simulink model "IEEE39bus"  (Simulink 8.5)
settings: Solver=ode3  SolverMode=SingleTasking  StartTime=0.0  StopTime=50  FixedStep=Ts  RelTol=1e-3
PostLoadFcn:
  | Ts=25e-6; IEEE39BusLineLength;
  | vNomHV = 345E3;fNom=50;load('Dynamicload.mat');
InitFcn:
  | Ts=25e-6; IEEE39BusLineLength;
  | vNomHV = 345E3;fNom=50;load('Dynamicload.mat');
undefined symbols (not defined in the file): D1, Delta, load15, load16, load18, load20, load21, load23, load24, load25, load26, load27, load28, load29, load3, load39, load4, load7, load8, TL_10_11_len, TL_10_13_len, TL_13_14_len, TL_14_15_len, TL_15_16_len, TL_16_17_len, TL_16_19_len, TL_16_21_len, TL_16_24_len, TL_17_18_len, TL_17_27_len, TL_1_2_len, TL_1_39_len, TL_21_22_len, TL_22_23_len, TL_24_23_len, TL_25_26_len, TL_26_27_len, TL_26_28_len, TL_26_29_len, TL_28_29_len, TL_2_25_len, TL_2_2_len, TL_3_18_len, TL_3_4_len, TL_4_14_len, TL_4_5_len, TL_5_6_len, TL_5_8_len, TL_6_11_len, TL_6_7_len, TL_7_8_len, TL_8_9_len, TL_9_39_len
libraries: powerlib x175, op_dpl_lib x34, rtlab x14, sps_avr x9, powerlib_extras x2, artemis x1, powerlib_meascontrol x1
(part 4 of 5)

== system IEEE39bus/SS_WestSystem1/GT 1  ==
  The Electric Power Grid : Subsystem  mask(The Electric Power Grid){pTotal=3, fNom=50, vNom=22e3*(1E-3)*1.05, pFeeder=185.5-50}
      mask prompts: pTotal "Total grid generation (GWatt)"; fNom "Nominal frequency (Hz)"; vNom "Nominal L-L voltage (kV)"; pFeeder "Initial feeder consumption (MWatt)"
      mask init:
      | % this is a patch for Simulink limitation on expression evaluation at model
      | % opening to avoid a error message
      | initPm0=(0.7*pTotal*1E9+pFeeder*1E6+1E6)/(pTotal*1E9);
      mask Display: image(imread('EPG.jpg'))
  A : PMIOPort  Port=1  Side=Right
  B : PMIOPort  Port=2  Side=Right
  C : PMIOPort  Port=3  Side=Right
  tag scope: V_G1=global
  wires:
  [V_bus_G1] -> [V_G1]
  connections:
  The Electric Power Grid/RConn3 -- C/RConn1
  B/RConn1 -- The Electric Power Grid/RConn2
  A/RConn1 -- The Electric Power Grid/RConn1

== system IEEE39bus/SS_WestSystem1/Load 39 ==
  Bus_L39 : powerlib/Measurements/Three-Phase V-I Measurement  VoltageMeasurement=phase-to-ground  SetLabelV=off  LabelV=V_Bus_L39  Vpu=off  VpuLL=off  CurrentMeasurement=yes  SetLabelI=on  LabelI=I_L39  Ipu=off  Pbase=100e6  Vbase=230e3  OutputType=Complex  PhasorSimulation=off  PSBequivalent=0
  Terminator : Terminator
  Three-Phase Dynamic Load : powerlib/Elements/Three-Phase Dynamic Load  NominalVoltage=[345e3 50 ]  ActiveReactivePowers=[1.104e+09 2.5e+08]  PositiveSequence=[1.02945 21.8447]  ExternalControl=on  NpNq=[0 0]  TimeConstants="[0  0  0  0]"  MinimumVoltage=0.7  LoadFlowParameters=[4,0,0,0,0]
  A : PMIOPort  Port=1  Side=Left
  B : PMIOPort  Port=2  Side=Left
  C : PMIOPort  Port=3  Side=Left
  tag scope: V_L39=global
  wires:
  Three-Phase Dynamic Load/1 -> Terminator/1
  Bus_L39/1 -> [V_L39]
  [load39] -> Three-Phase Dynamic Load/1
  connections:
  Three-Phase Dynamic Load/LConn1 -- Bus_L39/RConn1
  C/RConn1 -- Bus_L39/LConn3
  B/RConn1 -- Bus_L39/LConn2
  A/RConn1 -- Bus_L39/LConn1
  Bus_L39/RConn2 -- Three-Phase Dynamic Load/LConn2
  Bus_L39/RConn3 -- Three-Phase Dynamic Load/LConn3

== system IEEE39bus/SS_WestSystem1/Load 4 ==
  Bus_L4 : powerlib/Measurements/Three-Phase V-I Measurement  VoltageMeasurement=phase-to-ground  SetLabelV=off  LabelV=V_Bus_L4  Vpu=off  VpuLL=off  CurrentMeasurement=yes  SetLabelI=on  LabelI=I_L4  Ipu=off  Pbase=100e6  Vbase=230e3  OutputType=Complex  PhasorSimulation=off  PSBequivalent=0
  Terminator : Terminator
  Three-Phase Dynamic Load : powerlib/Elements/Three-Phase Dynamic Load  NominalVoltage=[ 345e3 50 ]  ActiveReactivePowers=[5e+08 1.84e+08]  PositiveSequence=[0.993488 19.1617]  ExternalControl=on  NpNq=[0 0]  TimeConstants="[0  0  0  0]"  MinimumVoltage=0.7  LoadFlowParameters=[4,0,0,0,0]
  A : PMIOPort  Port=1  Side=Left
  B : PMIOPort  Port=2  Side=Left
  C : PMIOPort  Port=3  Side=Left
  tag scope: V_L4=global
  wires:
  Three-Phase Dynamic Load/1 -> Terminator/1
  Bus_L4/1 -> [V_L4]
  [load4] -> Three-Phase Dynamic Load/1
  connections:
  Three-Phase Dynamic Load/LConn3 -- Bus_L4/RConn3
  Three-Phase Dynamic Load/LConn2 -- Bus_L4/RConn2
  A/RConn1 -- Bus_L4/LConn1
  B/RConn1 -- Bus_L4/LConn2
  C/RConn1 -- Bus_L4/LConn3
  Three-Phase Dynamic Load/LConn1 -- Bus_L4/RConn1

== system IEEE39bus/SS_WestSystem1/Load 8 ==
  Bus_L8 : powerlib/Measurements/Three-Phase V-I Measurement  VoltageMeasurement=phase-to-ground  SetLabelV=off  LabelV=V_Bus_L8  Vpu=off  VpuLL=off  CurrentMeasurement=yes  SetLabelI=on  LabelI=I_L8  Ipu=off  Pbase=100e6  Vbase=230e3  OutputType=Complex  PhasorSimulation=off  PSBequivalent=0
  Terminator : Terminator
  Three-Phase Dynamic Load : powerlib/Elements/Three-Phase Dynamic Load  NominalVoltage=[345e3 50 ]  ActiveReactivePowers=[5.22e+08 1.76e+08]  PositiveSequence=[0.991583 18.8054]  ExternalControl=on  NpNq=[0 0]  TimeConstants="[0  0  0  0]"  MinimumVoltage=0.7  LoadFlowParameters=[4,0,0,0,0]
  A : PMIOPort  Port=1  Side=Left
  B : PMIOPort  Port=2  Side=Left
  C : PMIOPort  Port=3  Side=Left
  tag scope: V_L8=global
  wires:
  Three-Phase Dynamic Load/1 -> Terminator/1
  Bus_L8/1 -> [V_L8]
  [load8] -> Three-Phase Dynamic Load/1
  connections:
  Three-Phase Dynamic Load/LConn1 -- Bus_L8/RConn1
  C/RConn1 -- Bus_L8/LConn3
  B/RConn1 -- Bus_L8/LConn2
  A/RConn1 -- Bus_L8/LConn1
  Three-Phase Dynamic Load/LConn2 -- Bus_L8/RConn2
  Three-Phase Dynamic Load/LConn3 -- Bus_L8/RConn3

== system IEEE39bus/SS_WestSystem1/Machines Measurements ==
  Mux1 : Mux
  Machines Measurements : Outport
  wires:
  Mux1/1 -> Machines Measurements/1
  [Wm_G1] -> Mux1/4
  [Q_G1] -> Mux1/3
  [P_G1] -> Mux1/2
  [V_G1] -> Mux1/1

== system IEEE39bus/SS_WestSystem2/Buses Current_W ==
  Mux3 : Mux  Inputs=6
  Current : Outport
  wires:
  Mux3/1 -> Current/1
  [I_bus_6] -> Mux3/1
  [I_L7] -> Mux3/2
  [I_bus_13] -> Mux3/6
  [I_L12] -> Mux3/5
  [I_bus_11] -> Mux3/4
  [I_bus_10] -> Mux3/3

== system IEEE39bus/SS_WestSystem2/Buses voltages_W ==
  Mux3 : Mux  Inputs=6
  Voltages : Outport
  wires:
  [V_L7] -> Mux3/2
  [V_bus_10] -> Mux3/3
  [V_L12] -> Mux3/5
  [V_bus_11] -> Mux3/4
  [V_bus_13] -> Mux3/6
  [V_bus_6] -> Mux3/1
  Mux3/1 -> Voltages/1

== system IEEE39bus/SS_WestSystem2/GT 2- Slack ==
  5 MW : powerlib/Elements/Three-Phase Parallel RLC Load  LConnTagsString=A|B|C  Configuration=Y (grounded)  NominalVoltage=22e3  NominalFrequency=50  ActivePower=5e6  InductivePower=0  CapacitivePower=0  Measurements=None  LoadType=constant Z
  Bus Selector1 : BusSelector  OutputSignals="dq0 components.Stator voltage  vq (pu),dq0 components.Stator voltage  vd (pu),Mechanical.Rotor speed  wm  (pu),Mechanical.Rotor speed deviation  dw (pu),Output active power   Peo (pu),Output reactive power  Qeo (pu)"
  Bus 31 : powerlib/Measurements/Three-Phase V-I Measurement  VoltageMeasurement=phase-to-ground  SetLabelV=on  LabelV=V_bus_G2  Vpu=off  VpuLL=off  CurrentMeasurement=no  SetLabelI=on  LabelI=I_bus_G2  Ipu=off  Pbase=100e6  Vbase=16.5e3  OutputType=Complex  PhasorSimulation=off  PSBequivalent=0
  Excitation System : sps_avr/Excitation System  tr=20e-3  reg=[ 200, 0.02 ]  exc=[ 1, 0 .19]  tgr=[ 0, 0 ]  damp=[ 0.0012, 1 ]  sat=[ 0, 0 ]  lim=[ 0, 7.32, 0 ]  v0=[0.982 2.0635]
  GT1_CB2 : Subsystem
  Ground : Ground
  HTG : powerlib/Machines/Hydraulic Turbine and Governor  sm="[ 10/3  0.07 ]"  gate="[  0.01  0.97518  -0.1  0.1 ]"  reg="[  0.05  1.163  0.105  0  0.01  ]"  hyd="[  0  2.67  ]"  dref=0  po=0.84
  Load 31 : Subsystem
  Load Flow Bus : powerlib/Measurements/Load Flow Bus  LConnTagsString=a  ID=Bus-31  Vbase=22000  Vref=0.982  Vangle=0  VLF=0.982  angleLF=0
      settings: AttributesFormatString=%<ID>\n%<Vbase>V\n%<VLF>pu\n%<angleLF>deg.
  Machine 2 1000 MVA 22 kV : powerlib/Machines/Synchronous Machine pu Standard  PresetModel=No  MechanicalLoad=Mechanical power Pm  ShowDetailedParameters=on  RotorType=Round  Units=per unit standard parameters  MeasurementBus=off  NominalParameters=[1000e+006 22000 50]  Reactances1=[ 1.693 0.4 0.2 1.618 0.967 0.2 0.035 ]  Reactances2=[1.699 0.174 0.109 0.838 0.185 0.069]  dAxisTimeConstants=Open-circuit  qAxisTimeConstants=Open-circuit  TimeConstants1=[]  TimeConstants2=[6.56 0.03 1.5 0.04]  TimeConstants3=[]  TimeConstants4=[]  TimeConstants5=[ 9.2, 0.01, 0.01 ]  TimeConstants6=[]  TimeConstants7=[0.024 0.006 0.006]  TimeConstants8=[1 2 3 1]  StatorResistance=0.005  Mechanical=[5.28 0.02558 2]  PolePairs=2  InitialConditions=[0 -44.333 0.922146 0.922146 0.922146 -16.0713 -136.071 103.929 2.06352]  SetSaturation=off  Saturation=[0.6404,0.7127,0.8441,0.9214,0.9956,1.082,1.19,1.316,1.457;0.7,0.7698,0.8872,0.9466,0.9969,1.046,1.1,1.151,1.201]  LoadFlowParameters=[1 524200000 21604 0]  TsPowergui=0  TsBlock=-1  IterativeModel=Trapezoidal non iterative  BusType=swing  Pref=5.242e+008  Qref=0  Qmin=-Inf  Qmax=Inf  PLF=0  QLF=0
      settings: AttributesFormatString=\n\n
  Pref : Constant  Value=0.84
  Terminator5 : Terminator
  Transformer 2 631.4 MVA 22 kV / 345 kV : powerlib/Elements/Three-Phase Transformer (Two Windings)  Winding1Connection=Delta (D1)  Winding2Connection=Yg  CoreType=Three single-phase transformers  SetSaturation=off  Hysteresis=off  DataFile='hysteresis'  SetInitialFlux=off  Measurements=None  UNITS=pu  NominalPower=[ 1000e+6 50 ]  Winding1="[ 22e3   0.0     0.025*1000/100/2]"  Winding2="[ 1.07*345e3  0.0     0.025*1000/100/2 ]"  Rm=500  Lm=500  L0=0.5  Saturation="[ 0,0  ;  0.005,1.2  ;  1.0,1.4 ]"  InitialFluxes=[ 0.8 , -0.8 , 0.7 ]  MoreParameters=off  BreakLoop=off  DataType=off  TransfoNumber=0
  Vref : Constant  Value=0.982
  wref : Constant
  A : PMIOPort  Port=1  Side=Right
  B : PMIOPort  Port=2  Side=Right
  C : PMIOPort  Port=3  Side=Right
  tag scope: P_G2=global, Q_G2=global, V_G2=global, Wm_G2=global
  wires:
  Ground/1 -> Excitation System/4
  HTG/2 -> Terminator5/1
  Vref/1 -> Excitation System/1
  Pref/1 -> HTG/2
  wref/1 -> HTG/1
  Excitation System/1 -> Machine 2 1000 MVA 22 kV/2
  HTG/1 -> Machine 2 1000 MVA 22 kV/1
  Machine 2 1000 MVA 22 kV/1 -> Bus Selector1/1
  Bus Selector1/1 -> Excitation System/3  "<Stator voltage  vq (pu)>"
  Bus Selector1/2 -> Excitation System/2  "<Stator voltage  vd (pu)>"
  Bus Selector1/3 -> HTG/3, [Wm_G2]  "<Rotor speed  wm  (pu)>"
  Bus Selector1/4 -> HTG/5  "<Rotor speed deviation  dw (pu)>"
  Bus Selector1/5 -> HTG/4, [P_G2]  "<Output active power   Peo (pu)>"
  Bus Selector1/6 -> [Q_G2]  "<Output reactive power  Qeo (pu)>"
  [V_bus_G2] -> [V_G2]
  connections:
  Bus 31/RConn1 -- Load 31/LConn1 -- Transformer 2 631.4 MVA 22 kV / 345 kV/LConn1 -- Load Flow Bus/LConn1 -- 5 MW/LConn1
  Load 31/LConn2 -- Bus 31/RConn2 -- Transformer 2 631.4 MVA 22 kV / 345 kV/LConn2 -- 5 MW/LConn2
  Load 31/LConn3 -- Bus 31/RConn3 -- Transformer 2 631.4 MVA 22 kV / 345 kV/LConn3 -- 5 MW/LConn3
  Machine 2 1000 MVA 22 kV/RConn1 -- Bus 31/LConn1
  Machine 2 1000 MVA 22 kV/RConn2 -- Bus 31/LConn2
  Machine 2 1000 MVA 22 kV/RConn3 -- Bus 31/LConn3
  GT1_CB2/LConn1 -- Transformer 2 631.4 MVA 22 kV / 345 kV/RConn1
  GT1_CB2/LConn2 -- Transformer 2 631.4 MVA 22 kV / 345 kV/RConn2
  GT1_CB2/LConn3 -- Transformer 2 631.4 MVA 22 kV / 345 kV/RConn3
  A/RConn1 -- GT1_CB2/RConn1
  C/RConn1 -- GT1_CB2/RConn3
  B/RConn1 -- GT1_CB2/RConn2

== system IEEE39bus/SS_WestSystem2/GT 3 ==
  5 MW : powerlib/Elements/Three-Phase Parallel RLC Load  LConnTagsString=A|B|C  Configuration=Y (grounded)  NominalVoltage=22e3  NominalFrequency=50  ActivePower=5e6  InductivePower=0  CapacitivePower=0  Measurements=None  LoadType=constant Z
  Bus Selector1 : BusSelector  OutputSignals="dq0 components.Stator voltage  vq (pu),dq0 components.Stator voltage  vd (pu),Mechanical.Rotor speed  wm  (pu),Mechanical.Rotor speed deviation  dw (pu),Output active power   Peo (pu),Output reactive power  Qeo (pu)"
  Bus 32 : powerlib/Measurements/Three-Phase V-I Measurement  VoltageMeasurement=phase-to-ground  SetLabelV=on  LabelV=V_bus_G3  Vpu=off  VpuLL=off  CurrentMeasurement=no  SetLabelI=on  LabelI=I_bus_G3  Ipu=off  Pbase=100e6  Vbase=16.5e3  OutputType=Complex  PhasorSimulation=off  PSBequivalent=0
  Excitation System : sps_avr/Excitation System  tr=20e-3  reg=[ 200, 0.02 ]  exc=[ 1, 0 .19]  tgr=[ 0, 0 ]  damp=[ 0.0012, 1 ]  sat=[ 0, 0 ]  lim=[ 0, 7.32, 0 ]  v0=[1 1.7514]
  GT1_CB3 : Subsystem
  Ground : Ground
  HTG : powerlib/Machines/Hydraulic Turbine and Governor  sm="[ 10/3  0.07 ]"  gate="[  0.01  0.97518  -0.1  0.1 ]"  reg="[  0.05  1.163  0.105  0  0.01  ]"  hyd="[  0  2.67  ]"  dref=0  po=0.525
  Load Flow Bus : powerlib/Measurements/Load Flow Bus  LConnTagsString=a  ID=Bus-32  Vbase=22000  Vref=1  Vangle=0  VLF=1  angleLF=-2.403
      settings: AttributesFormatString=%<ID>\n%<Vbase>V\n%<VLF>pu\n%<angleLF>deg.
  Machine 3 1000 MVA 22 kV : powerlib/Machines/Synchronous Machine pu Standard  PresetModel=No  MechanicalLoad=Mechanical power Pm  ShowDetailedParameters=on  RotorType=Round  Units=per unit standard parameters  MeasurementBus=off  NominalParameters="[ 1000E6  22000   50 ]"  Reactances1=[ 1.879 0.4 0.2 1.785 0.66 0.2 0.03 ]  Reactances2=[ 0.995, 0.195, 0.155, 0.568, 0.143, 0.16 ]  dAxisTimeConstants=Open-circuit  qAxisTimeConstants=Open-circuit  TimeConstants1=[]  TimeConstants2=[5.7 0.03 1.5 0.04]  TimeConstants3=[]  TimeConstants4=[]  TimeConstants5=[ 9.2, 0.01, 0.01 ]  TimeConstants6=[]  TimeConstants7=[]  TimeConstants8=[]  StatorResistance=0.005  Mechanical=[ 4.75 0.02 20]  PolePairs=20  InitialConditions=[0 -57.2872 0.592169 0.592169 0.592169 -24.1565 -144.157 95.8435 1.7514]  SetSaturation=off  Saturation=[0.6404,0.7127,0.8441,0.9214,0.9956,1.082,1.19,1.316,1.457;0.7,0.7698,0.8872,0.9466,0.9969,1.046,1.1,1.151,1.201]  LoadFlowParameters=[1 650000000 21628.2 0]  TsPowergui=0  TsBlock=-1  IterativeModel=Trapezoidal non iterative  BusType=PV  Pref=5.50e+008  Qref=0  Qmin=-500e6  Qmax=250e6  PLF=0  QLF=0
      settings: AttributesFormatString=\n\n
  Pref : Constant  Value=0.525
  Terminator5 : Terminator
  Transformer 3 828.3 MVA 22 kV / 345 kV : powerlib/Elements/Three-Phase Transformer (Two Windings)  Winding1Connection=Delta (D1)  Winding2Connection=Yg  CoreType=Three single-phase transformers  SetSaturation=off  Hysteresis=off  DataFile='hysteresis'  SetInitialFlux=off  Measurements=None  UNITS=pu  NominalPower=[ 1000e6 60 ]  Winding1="[ 22e3 0  0.02*1000/100/2]"  Winding2="[ 1.045*345e3  0  0.02*1000/100/2]"  Rm=500  Lm=500  L0=0.5  Saturation="[ 0,0  ;  0.005,1.2  ;  1.0,1.4 ]"  InitialFluxes=[ 0.8 , -0.8 , 0.7 ]  MoreParameters=off  BreakLoop=off  DataType=off  TransfoNumber=0
  Vref : Constant
  wref : Constant
  A : PMIOPort  Port=1  Side=Right
  B : PMIOPort  Port=2  Side=Right
  C : PMIOPort  Port=3  Side=Right
  tag scope: P_G3=global, Q_G3=global, V_G3=global, Wm_G3=global
  wires:
  Ground/1 -> Excitation System/4
  HTG/2 -> Terminator5/1
  Vref/1 -> Excitation System/1
  Pref/1 -> HTG/2
  wref/1 -> HTG/1
  Excitation System/1 -> Machine 3 1000 MVA 22 kV/2
  HTG/1 -> Machine 3 1000 MVA 22 kV/1
  Machine 3 1000 MVA 22 kV/1 -> Bus Selector1/1
  Bus Selector1/1 -> Excitation System/3  "<Stator voltage  vq (pu)>"
  Bus Selector1/2 -> Excitation System/2  "<Stator voltage  vd (pu)>"
  Bus Selector1/3 -> HTG/3, [Wm_G3]  "<Rotor speed  wm  (pu)>"
  Bus Selector1/4 -> HTG/5  "<Rotor speed deviation  dw (pu)>"
  Bus Selector1/5 -> HTG/4, [P_G3]  "<Output active power   Peo (pu)>"
  Bus Selector1/6 -> [Q_G3]  "<Output reactive power  Qeo (pu)>"
  [V_bus_G3] -> [V_G3]
  connections:
  Transformer 3 828.3 MVA 22 kV / 345 kV/LConn1 -- Load Flow Bus/LConn1 -- Bus 32/RConn1 -- 5 MW/LConn1
  Transformer 3 828.3 MVA 22 kV / 345 kV/LConn2 -- Bus 32/RConn2 -- 5 MW/LConn2
  Transformer 3 828.3 MVA 22 kV / 345 kV/LConn3 -- Bus 32/RConn3 -- 5 MW/LConn3
  Machine 3 1000 MVA 22 kV/RConn1 -- Bus 32/LConn1
  Machine 3 1000 MVA 22 kV/RConn2 -- Bus 32/LConn2
  Machine 3 1000 MVA 22 kV/RConn3 -- Bus 32/LConn3
  GT1_CB3/LConn1 -- Transformer 3 828.3 MVA 22 kV / 345 kV/RConn1
  GT1_CB3/LConn2 -- Transformer 3 828.3 MVA 22 kV / 345 kV/RConn2
  GT1_CB3/LConn3 -- Transformer 3 828.3 MVA 22 kV / 345 kV/RConn3
  B/RConn1 -- GT1_CB3/RConn2
  A/RConn1 -- GT1_CB3/RConn1
  C/RConn1 -- GT1_CB3/RConn3

== system IEEE39bus/SS_WestSystem2/Load 12 ==
  Bus_L12 : powerlib/Measurements/Three-Phase V-I Measurement  VoltageMeasurement=phase-to-ground  SetLabelV=off  LabelV=V_Bus_L12  Vpu=off  VpuLL=off  CurrentMeasurement=yes  SetLabelI=on  LabelI=I_L12  Ipu=off  Pbase=100e6  Vbase=230e3  OutputType=Complex  PhasorSimulation=off  PSBequivalent=0
  Snubber : powerlib/Elements/Three-Phase Series RLC Load  LConnTagsString=A|B|C  Configuration=Y (grounded)  NominalVoltage=345E3  NominalFrequency=50  ActivePower=1e6  InductivePower=0  CapacitivePower=1e7  Measurements=None  LoadType=constant Z
  Terminator : Terminator
  Three-Phase Dynamic Load : powerlib/Elements/Three-Phase Dynamic Load  NominalVoltage=[345e3 50 ]  ActiveReactivePowers=[7.5e+06 8.8e+07]  PositiveSequence=[0.996047 51.6025]  ExternalControl=off  NpNq=[0 0]  TimeConstants="[0  0  0  0]"  MinimumVoltage=0.7  LoadFlowParameters=[4,0,0,0,0]
  A : PMIOPort  Port=1  Side=Left
  B : PMIOPort  Port=2  Side=Left
  C : PMIOPort  Port=3  Side=Left
  tag scope: V_L12=global
  wires:
  Three-Phase Dynamic Load/1 -> Terminator/1
  Bus_L12/1 -> [V_L12]
  connections:
  Snubber/LConn1 -- Bus_L12/RConn1 -- Three-Phase Dynamic Load/LConn1
  C/RConn1 -- Bus_L12/LConn3
  B/RConn1 -- Bus_L12/LConn2
  A/RConn1 -- Bus_L12/LConn1
  Bus_L12/RConn2 -- Snubber/LConn2 -- Three-Phase Dynamic Load/LConn2
  Snubber/LConn3 -- Bus_L12/RConn3 -- Three-Phase Dynamic Load/LConn3

== system IEEE39bus/SS_WestSystem2/Load 7 ==
  Bus_L7 : powerlib/Measurements/Three-Phase V-I Measurement  VoltageMeasurement=phase-to-ground  SetLabelV=off  LabelV=V_Bus_L7  Vpu=off  VpuLL=off  CurrentMeasurement=yes  SetLabelI=on  LabelI=I_L7  Ipu=off  Pbase=100e6  Vbase=230e3  OutputType=Complex  PhasorSimulation=off  PSBequivalent=0
  Terminator : Terminator
  Three-Phase Dynamic Load : powerlib/Elements/Three-Phase Dynamic Load  NominalVoltage=[ 345e3 50]  ActiveReactivePowers=[2.338e+08 8.4e+07]  PositiveSequence=[0.992793 19.1857]  ExternalControl=on  NpNq=[0 0]  TimeConstants="[0  0  0  0]"  MinimumVoltage=0.7  LoadFlowParameters=[4,0,0,0,0]
  A : PMIOPort  Port=1  Side=Left
  B : PMIOPort  Port=2  Side=Left
  C : PMIOPort  Port=3  Side=Left
  tag scope: V_L7=global
  wires:
  Three-Phase Dynamic Load/1 -> Terminator/1
  Bus_L7/1 -> [V_L7]
  [load7] -> Three-Phase Dynamic Load/1
  connections:
  Bus_L7/RConn3 -- Three-Phase Dynamic Load/LConn3
  Bus_L7/RConn2 -- Three-Phase Dynamic Load/LConn2
  A/RConn1 -- Bus_L7/LConn1
  B/RConn1 -- Bus_L7/LConn2
  C/RConn1 -- Bus_L7/LConn3
  Bus_L7/RConn1 -- Three-Phase Dynamic Load/LConn1

== system IEEE39bus/SS_WestSystem2/Machines Measurements ==
  Mux : Mux  Inputs=2
  Mux2 : Mux
  Mux3 : Mux
  Machines Measurements : Outport
  wires:
  [Wm_G3] -> Mux3/4
  [Q_G3] -> Mux3/3
  [P_G3] -> Mux3/2
  [V_G3] -> Mux3/1
  Mux2/1 -> Mux/1
  Mux/1 -> Machines Measurements/1
  [Wm_G2] -> Mux2/4
  [Q_G2] -> Mux2/3
  [P_G2] -> Mux2/2
  [V_G2] -> Mux2/1
  Mux3/1 -> Mux/2

== system IEEE39bus/SS_EastSystem1/GT 4/GT1_CB4 ==
  GT1_CB : powerlib/Elements/Three-Phase Breaker  InitialState=closed  SwitchA=on  SwitchB=on  SwitchC=on  SwitchTimes=[15]  External=on  BreakerResistance=0.001  SnubberResistance=1e6  SnubberCapacitance=inf  Measurements=None
  Cnn1 : PMIOPort  Port=1  Side=Right
  Conn2 : PMIOPort  Port=2  Side=Left
  Conn3 : PMIOPort  Port=3  Side=Right
  Conn4 : PMIOPort  Port=4  Side=Left
  Conn5 : PMIOPort  Port=5  Side=Left
  Conn6 : PMIOPort  Port=6  Side=Right
  wires:
  [GT4_CB] -> GT1_CB/1
  connections:
  Cnn1/RConn1 -- GT1_CB/RConn1
  Conn2/RConn1 -- GT1_CB/LConn1
  Conn3/RConn1 -- GT1_CB/RConn2
  Conn4/RConn1 -- GT1_CB/LConn2
  Conn5/RConn1 -- GT1_CB/LConn3
  Conn6/RConn1 -- GT1_CB/RConn3

== system IEEE39bus/SS_EastSystem1/GT 5/GT1_CB6 ==
  GT1_CB : powerlib/Elements/Three-Phase Breaker  InitialState=closed  SwitchA=on  SwitchB=on  SwitchC=on  SwitchTimes=[15]  External=on  BreakerResistance=0.001  SnubberResistance=1e6  SnubberCapacitance=inf  Measurements=None
  Cnn1 : PMIOPort  Port=1  Side=Right
  Conn2 : PMIOPort  Port=2  Side=Left
  Conn3 : PMIOPort  Port=3  Side=Right
  Conn4 : PMIOPort  Port=4  Side=Left
  Conn5 : PMIOPort  Port=5  Side=Left
  Conn6 : PMIOPort  Port=6  Side=Right
  wires:
  [GT5_CB] -> GT1_CB/1
  connections:
  Cnn1/RConn1 -- GT1_CB/RConn1
  Conn2/RConn1 -- GT1_CB/LConn1
  Conn3/RConn1 -- GT1_CB/RConn2
  Conn4/RConn1 -- GT1_CB/LConn2
  Conn5/RConn1 -- GT1_CB/LConn3
  Conn6/RConn1 -- GT1_CB/RConn3

== system IEEE39bus/SS_EastSystem2/GT 6/GT1_CB8 ==
  GT1_CB : powerlib/Elements/Three-Phase Breaker  InitialState=closed  SwitchA=on  SwitchB=on  SwitchC=on  SwitchTimes=[15]  External=on  BreakerResistance=0.001  SnubberResistance=1e6  SnubberCapacitance=inf  Measurements=None
  Cnn1 : PMIOPort  Port=1  Side=Right
  Conn2 : PMIOPort  Port=2  Side=Left
  Conn3 : PMIOPort  Port=3  Side=Right
  Conn4 : PMIOPort  Port=4  Side=Left
  Conn5 : PMIOPort  Port=5  Side=Left
  Conn6 : PMIOPort  Port=6  Side=Right
  wires:
  [GT6_CB] -> GT1_CB/1
  connections:
  Cnn1/RConn1 -- GT1_CB/RConn1
  Conn2/RConn1 -- GT1_CB/LConn1
  Conn3/RConn1 -- GT1_CB/RConn2
  Conn4/RConn1 -- GT1_CB/LConn2
  Conn5/RConn1 -- GT1_CB/LConn3
  Conn6/RConn1 -- GT1_CB/RConn3

== system IEEE39bus/SS_EastSystem2/GT 7/GT1_CB10 ==
  GT1_CB : powerlib/Elements/Three-Phase Breaker  InitialState=closed  SwitchA=on  SwitchB=on  SwitchC=on  SwitchTimes=[15]  External=on  BreakerResistance=0.001  SnubberResistance=1e6  SnubberCapacitance=inf  Measurements=None
  Cnn1 : PMIOPort  Port=1  Side=Right
  Conn2 : PMIOPort  Port=2  Side=Left
  Conn3 : PMIOPort  Port=3  Side=Right
  Conn4 : PMIOPort  Port=4  Side=Left
  Conn5 : PMIOPort  Port=5  Side=Left
  Conn6 : PMIOPort  Port=6  Side=Right
  wires:
  [GT7_CB] -> GT1_CB/1
  connections:
  Cnn1/RConn1 -- GT1_CB/RConn1
  Conn2/RConn1 -- GT1_CB/LConn1
  Conn3/RConn1 -- GT1_CB/RConn2
  Conn4/RConn1 -- GT1_CB/LConn2
  Conn5/RConn1 -- GT1_CB/LConn3
  Conn6/RConn1 -- GT1_CB/RConn3

== system IEEE39bus/SS_NorthSystem1/GT 8/GT1_CB11 ==
  GT1_CB : powerlib/Elements/Three-Phase Breaker  InitialState=closed  SwitchA=on  SwitchB=on  SwitchC=on  SwitchTimes=[15]  External=on  BreakerResistance=0.001  SnubberResistance=1e6  SnubberCapacitance=inf  Measurements=None
  Cnn1 : PMIOPort  Port=1  Side=Right
  Conn2 : PMIOPort  Port=2  Side=Left
  Conn3 : PMIOPort  Port=3  Side=Right
  Conn4 : PMIOPort  Port=4  Side=Left
  Conn5 : PMIOPort  Port=5  Side=Left
  Conn6 : PMIOPort  Port=6  Side=Right
  wires:
  [GT8_CB] -> GT1_CB/1
  connections:
  Cnn1/RConn1 -- GT1_CB/RConn1
  Conn2/RConn1 -- GT1_CB/LConn1
  Conn3/RConn1 -- GT1_CB/RConn2
  Conn4/RConn1 -- GT1_CB/LConn2
  Conn5/RConn1 -- GT1_CB/LConn3
  Conn6/RConn1 -- GT1_CB/RConn3

== system IEEE39bus/SS_NorthSystem1/GT 9/GT1_CB12 ==
  GT1_CB : powerlib/Elements/Three-Phase Breaker  InitialState=closed  SwitchA=on  SwitchB=on  SwitchC=on  SwitchTimes=[15]  External=on  BreakerResistance=0.001  SnubberResistance=1e6  SnubberCapacitance=inf  Measurements=None
  Cnn1 : PMIOPort  Port=1  Side=Right
  Conn2 : PMIOPort  Port=2  Side=Left
  Conn3 : PMIOPort  Port=3  Side=Right
  Conn4 : PMIOPort  Port=4  Side=Left
  Conn5 : PMIOPort  Port=5  Side=Left
  Conn6 : PMIOPort  Port=6  Side=Right
  wires:
  [GT9_CB] -> GT1_CB/1
  connections:
  Cnn1/RConn1 -- GT1_CB/RConn1
  Conn2/RConn1 -- GT1_CB/LConn1
  Conn3/RConn1 -- GT1_CB/RConn2
  Conn4/RConn1 -- GT1_CB/LConn2
  Conn5/RConn1 -- GT1_CB/LConn3
  Conn6/RConn1 -- GT1_CB/RConn3

== system IEEE39bus/SS_NorthSystem2/GT 10/GT1_CB14 ==
  GT1_CB : powerlib/Elements/Three-Phase Breaker  InitialState=closed  SwitchA=on  SwitchB=on  SwitchC=on  SwitchTimes=[15]  External=on  BreakerResistance=0.001  SnubberResistance=1e6  SnubberCapacitance=inf  Measurements=None
  Cnn1 : PMIOPort  Port=1  Side=Right
  Conn2 : PMIOPort  Port=2  Side=Left
  Conn3 : PMIOPort  Port=3  Side=Right
  Conn4 : PMIOPort  Port=4  Side=Left
  Conn5 : PMIOPort  Port=5  Side=Left
  Conn6 : PMIOPort  Port=6  Side=Right
  wires:
  [GT10_CB] -> GT1_CB/1
  connections:
  Cnn1/RConn1 -- GT1_CB/RConn1
  Conn2/RConn1 -- GT1_CB/LConn1
  Conn3/RConn1 -- GT1_CB/RConn2
  Conn4/RConn1 -- GT1_CB/LConn2
  Conn5/RConn1 -- GT1_CB/LConn3
  Conn6/RConn1 -- GT1_CB/RConn3

== system IEEE39bus/SS_WestSystem1/GT 1 /The Electric Power Grid ==
  5 MW : powerlib/Elements/Three-Phase Parallel RLC Load  LConnTagsString=A|B|C  Configuration=Y (grounded)  NominalVoltage=345e3  NominalFrequency=50  ActivePower=5e6  InductivePower=0  CapacitivePower=0  Measurements=None  LoadType=constant Z
  Bus 39G : powerlib/Measurements/Three-Phase V-I Measurement  VoltageMeasurement=phase-to-ground  SetLabelV=on  LabelV=V_bus_G1  Vpu=off  VpuLL=off  CurrentMeasurement=no  SetLabelI=off  LabelI=I_bus_39  Ipu=off  Pbase=100e6  Vbase=345e3  OutputType=Complex  PhasorSimulation=off  PSBequivalent=0
  GT1_CB : Subsystem
  Load Flow Bus8 : powerlib/Measurements/Load Flow Bus  LConnTagsString=a  ID=Bus-39G  Vbase=22000  Vref=1.025  Vangle=0  VLF=1.025  angleLF=5.288
      settings: AttributesFormatString=%<ID>\n%<Vbase>V\n%<VLF>pu\n%<angleLF>deg.
  M1TurbineRegulators : Subsystem
  Memory : Memory
  Pref1 : Constant  Value=0.47
  Snubber : powerlib/Elements/Three-Phase Series RLC Load  LConnTagsString=A|B|C  Configuration=Y (grounded)  NominalVoltage=vNom*1E3  NominalFrequency=fNom  ActivePower=1e6  InductivePower=0  CapacitivePower=1e7  Measurements=None  LoadType=constant Z
  Synch : powerlib/Machines/Synchronous Machine pu Standard  PresetModel=No  MechanicalLoad=Mechanical power Pm  ShowDetailedParameters=on  RotorType=Round  Units=per unit standard parameters  MeasurementBus=off  NominalParameters="[pTotal*1E9  vNom*1E3   fNom ]"  Reactances1=[1.8 .3 .25 1.7 .55 .25 .2]  Reactances2=[ 1.305, 0.296, 0.252, 0.474, 0.243, 0.18 ]  dAxisTimeConstants=Open-circuit  qAxisTimeConstants=Open-circuit  TimeConstants1=[]  TimeConstants2=[8 .03 .4 .05]  TimeConstants3=[]  TimeConstants4=[]  TimeConstants5=[ 1.01, 0.053, 0.1 ]  TimeConstants6=[]  TimeConstants7=[]  TimeConstants8=[]  StatorResistance=0.0025  Mechanical="[ 6.5 0  4]"  PolePairs=4  InitialConditions=[0 -56.4125 0.421834 0.421834 0.421834 -16.137 -136.137 103.863 1.43951]  SetSaturation=off  Saturation=[0.6404,0.7127,0.8441,0.9214,0.9956,1.082,1.19,1.316,1.457;0.7,0.7698,0.8872,0.9466,0.9969,1.046,1.1,1.151,1.201]  LoadFlowParameters=[1 700000000 0 0 0]  TsPowergui=0  TsBlock=-1  IterativeModel=Forward Euler  BusType=PV  Pref=12e+8  Qref=0  Qmin=-inf  Qmax=inf  PLF=0  QLF=0
      settings: AttributesFormatString=\n\n
  Terminator : Terminator
  Transformer 3 2000 MVA 22 kV / 345 kV : powerlib/Elements/Three-Phase Transformer (Two Windings)  Winding1Connection=Delta (D1)  Winding2Connection=Yg  CoreType=Three single-phase transformers  SetSaturation=off  Hysteresis=off  DataFile='hysteresis'  SetInitialFlux=off  Measurements=None  UNITS=pu  NominalPower=[ 3000e6 50]  Winding1="[ 22e3 0  0.02*3000/100/2]"  Winding2="[ 1.07*345e3  0  0.02*3000/100/2]"  Rm=500  Lm=500  L0=0.5  Saturation="[ 0,0  ;  0.005,1.2  ;  1.0,1.4 ]"  InitialFluxes=[ 0.8 , -0.8 , 0.7 ]  MoreParameters=off  BreakLoop=off  DataType=off  TransfoNumber=0
  Vref1 : Constant  Value=0.97619
  A : PMIOPort  Tag=PMCPort  Port=1  Side=Right
  B : PMIOPort  Tag=PMCPort  Port=2  Side=Right
  C : PMIOPort  Tag=PMCPort  Port=3  Side=Right
  wires:
  Memory/1 -> M1TurbineRegulators/1(m)
  Synch/1 -> Memory/1
  M1TurbineRegulators/2(Vf) -> Synch/2
  M1TurbineRegulators/1(Pm) -> Synch/1
  Vref1/1 -> M1TurbineRegulators/3(Vref)
  Pref1/1 -> M1TurbineRegulators/2(Pref)
  M1TurbineRegulators/3(Peo_Delta) -> Terminator/1
  connections:
  Snubber/LConn1 -- Bus 39G/LConn1 -- Synch/RConn1
  Snubber/LConn2 -- Bus 39G/LConn2 -- Synch/RConn2
  Snubber/LConn3 -- Bus 39G/LConn3 -- Synch/RConn3
  Bus 39G/RConn1 -- 5 MW/LConn1 -- Transformer 3 2000 MVA 22 kV / 345 kV/LConn1
  Bus 39G/RConn2 -- 5 MW/LConn2 -- Transformer 3 2000 MVA 22 kV / 345 kV/LConn2
  Bus 39G/RConn3 -- Load Flow Bus8/LConn1 -- Transformer 3 2000 MVA 22 kV / 345 kV/LConn3 -- 5 MW/LConn3
  Transformer 3 2000 MVA 22 kV / 345 kV/RConn1 -- GT1_CB/LConn1
  Transformer 3 2000 MVA 22 kV / 345 kV/RConn3 -- GT1_CB/LConn3
  Transformer 3 2000 MVA 22 kV / 345 kV/RConn2 -- GT1_CB/LConn2
  C/RConn1 -- GT1_CB/RConn3
  B/RConn1 -- GT1_CB/RConn2
  A/RConn1 -- GT1_CB/RConn1

== system IEEE39bus/SS_WestSystem2/GT 2- Slack/GT1_CB2 ==
  GT1_CB : powerlib/Elements/Three-Phase Breaker  InitialState=closed  SwitchA=on  SwitchB=on  SwitchC=on  SwitchTimes=[15]  External=on  BreakerResistance=0.001  SnubberResistance=1e6  SnubberCapacitance=inf  Measurements=None
  Cnn1 : PMIOPort  Port=1  Side=Right
  Conn2 : PMIOPort  Port=2  Side=Left
  Conn3 : PMIOPort  Port=3  Side=Right
  Conn4 : PMIOPort  Port=4  Side=Left
  Conn5 : PMIOPort  Port=5  Side=Left
  Conn6 : PMIOPort  Port=6  Side=Right
  wires:
  [GT2_CB] -> GT1_CB/1
  connections:
  Cnn1/RConn1 -- GT1_CB/RConn1
  Conn2/RConn1 -- GT1_CB/LConn1
  Conn3/RConn1 -- GT1_CB/RConn2
  Conn4/RConn1 -- GT1_CB/LConn2
  Conn5/RConn1 -- GT1_CB/LConn3
  Conn6/RConn1 -- GT1_CB/RConn3

== system IEEE39bus/SS_WestSystem2/GT 2- Slack/Load 31 ==
  Bus_L29 : powerlib/Measurements/Three-Phase V-I Measurement  VoltageMeasurement=phase-to-ground  SetLabelV=off  LabelV=V_Bus_L29  Vpu=off  VpuLL=off  CurrentMeasurement=no  SetLabelI=on  LabelI=I_L10  Ipu=off  Pbase=100e6  Vbase=230e3  OutputType=Complex  PhasorSimulation=off  PSBequivalent=0
  Load 31 : Subsystem
  Terminator : Terminator
  Three-Phase Dynamic Load : powerlib/Elements/Three-Phase Dynamic Load  NominalVoltage=[345e3 50 ]  ActiveReactivePowers=[2.835e+08 2.69e+07]  PositiveSequence=[0.0626203 0]  ExternalControl=on  NpNq=[1.3 2]  TimeConstants="[0  0  0  0]"  MinimumVoltage=0.7  LoadFlowParameters=[4,0,0,0,0]
  A : PMIOPort  Port=1  Side=Left
  B : PMIOPort  Port=2  Side=Left
  C : PMIOPort  Port=3  Side=Left
  wires:
  Load 31/1(Load Power) -> Three-Phase Dynamic Load/1
  Three-Phase Dynamic Load/1 -> Terminator/1
  Bus_L29/1 -> Load 31/1(Vabc)
  connections:
  Three-Phase Dynamic Load/LConn1 -- Bus_L29/RConn1
  C/RConn1 -- Bus_L29/LConn3
  B/RConn1 -- Bus_L29/LConn2
  A/RConn1 -- Bus_L29/LConn1
  Bus_L29/RConn2 -- Three-Phase Dynamic Load/LConn2
  Bus_L29/RConn3 -- Three-Phase Dynamic Load/LConn3

== system IEEE39bus/SS_WestSystem2/GT 3/GT1_CB3 ==
  GT1_CB : powerlib/Elements/Three-Phase Breaker  InitialState=closed  SwitchA=on  SwitchB=on  SwitchC=on  SwitchTimes=[15]  External=on  BreakerResistance=0.001  SnubberResistance=1e6  SnubberCapacitance=inf  Measurements=None
  Cnn1 : PMIOPort  Port=1  Side=Right
  Conn2 : PMIOPort  Port=2  Side=Left
  Conn3 : PMIOPort  Port=3  Side=Right
  Conn4 : PMIOPort  Port=4  Side=Left
  Conn5 : PMIOPort  Port=5  Side=Left
  Conn6 : PMIOPort  Port=6  Side=Right
  wires:
  [GT3_CB] -> GT1_CB/1
  connections:
  Cnn1/RConn1 -- GT1_CB/RConn1
  Conn2/RConn1 -- GT1_CB/LConn1
  Conn3/RConn1 -- GT1_CB/RConn2
  Conn4/RConn1 -- GT1_CB/LConn2
  Conn5/RConn1 -- GT1_CB/LConn3
  Conn6/RConn1 -- GT1_CB/RConn3

== system IEEE39bus/SS_WestSystem1/GT 1 /The Electric Power Grid/GT1_CB ==
  GT1_CB : powerlib/Elements/Three-Phase Breaker  InitialState=closed  SwitchA=on  SwitchB=on  SwitchC=on  SwitchTimes=[15]  External=on  BreakerResistance=0.001  SnubberResistance=1e6  SnubberCapacitance=inf  Measurements=None
  Cnn1 : PMIOPort  Port=1  Side=Right
  Conn2 : PMIOPort  Port=2  Side=Left
  Conn3 : PMIOPort  Port=3  Side=Right
  Conn4 : PMIOPort  Port=4  Side=Left
  Conn5 : PMIOPort  Port=5  Side=Left
  Conn6 : PMIOPort  Port=6  Side=Right
  wires:
  [GT1_CB] -> GT1_CB/1
  connections:
  Cnn1/RConn1 -- GT1_CB/RConn1
  Conn2/RConn1 -- GT1_CB/LConn1
  Conn3/RConn1 -- GT1_CB/RConn2
  Conn4/RConn1 -- GT1_CB/LConn2
  Conn5/RConn1 -- GT1_CB/LConn3
  Conn6/RConn1 -- GT1_CB/RConn3

== system IEEE39bus/SS_WestSystem1/GT 1 /The Electric Power Grid/M1TurbineRegulators ==
  note: note: initial power of STG is modified automatically by upper Simulink mask
  m : Inport
  Pref : Inport  Port=2
  Vref : Inport  Port=3
  Bus Selector : BusSelector  OutputSignals="dq0 components.Stator voltage  vd (pu),dq0 components.Stator voltage  vq (pu),Mechanical.Rotor angle deviation  d_theta (rad),Mechanical.Rotor speed  wm  (pu),Mechanical.Rotor speed deviation  dw (pu),Load angle   delta  (deg),Output active power   Peo (pu),Output reactive power  Qeo (pu)"
  "Delta w PSS (Kundur) " : Subsystem  mask(Generic Power System Stabilizer){Tsensor=15e-3, K=30, Twashout=10, Tleadlag1=[50e-3 20e-3], Tleadlag2=[3 5.4], VSlimits=[-0.15 0.15], Vinit=0, Plot_On=off, MagdB_On=off, FreqRange=logspace(-2,2,500), Ts=Ts}
      mask prompts: Tsensor "Sensor time constant:"; K "Gain:"; Twashout "Wash-out time constant:"; Tleadlag1 "Lead-lag #1 time constants: [ Tnum Tden ]"; Tleadlag2 "Leag-lag #2 time constants: [ Tnum Tden ]"; VSlimits "Output limits: [ VSmin VSmax ]"; Vinit "Initial input:"; Plot_On "Plot frequency response"; MagdB_On "Magnitude in dB"; FreqRange "Frequency range (Hz):"; Ts "Sample Time"
      mask help:
      | This block implements a generic Power System Stabilizer (PSS). It consists of a
      | low-pass filter, a general gain, a washout high-pass filter, a phase-compensation
      | system, and an output limiter.
      |
      | The input is the synchronous machine speed deviation with respect to nominal
      | (dw in pu) or the acceleration power (Pa=Pm-Pe in pu).
      |
      | The output is the stabilization voltage, in p.u.
      mask init:
      | %powericon('psbcallbacks',gcb,'PSS',1);
      | T1n=Tleadlag1(1);
      | T1d=Tleadlag1(2);
      | T2n=Tleadlag2(1);
      | T2d=Tleadlag2(2);
      | %
      | if Plot_On==1,
      | % Compute global system (sysG):
      | numS=[1];
      | denS=[Tsensor 1];
      | sysS=tf(numS,denS);
      | numW=[Twashout 0];
      | denW=[Twashout 1];
      | sysW=tf(numW,denW);
      | numL1=[T1n 1];
      | denL1=[T1d 1];
      | sysL1=tf(numL1,denL1);
      | numL2=[T2n 1];
      | denL2=[T2d 1];
      | sysL2=tf(numL2,denL2);
      | sysG=sysS*K*sysW*sysL1*sysL2;
      | %
      | % Plot response:
      | w=2*pi*FreqRange;
      | [Mag,Pha]=bode(sysG,w);
      | subplot(2,1,1)
      | if  MagdB_On==1,
      | Y= 20*log10(squeeze(Mag)) ;
      | strLabel='dB';
      | else
      | Y=squeeze(Mag);
      | strLabel='pu/pu';
      | end
      | %
      | semilogx(FreqRange,Y)
      | ylabel(strLabel);grid;
      | title('PSS Frequency Response');
      | subplot(2,1,2);
      | semilogx(FreqRange,rem(squeeze(Pha),360))
      | ylabel('Degrees');grid;
      | xlabel('Frequency (Hz)');
      | end
      mask Help: web(psbhelp)
      mask Callback Plot_On: powericon('psbcallbacks',gcbh,'PSSmodel');
  EXCITATION : Subsystem  AncestorBlock=powerlib/Machines/Excitation System  mask(Excitation System){tr=20e-3, reg=[ 200, 0.001 ], exc=[ 1, 0 ], tgr=[ 0, 0 ], damp=[ 0, 0 ], sat=[ 0, 0 ], lim=[ 0 , 12.3, 0 ], v0=[0.97619 1.4395], Ts=Ts}
      mask prompts: tr "Low-pass filter time constant Tr(s):"; reg "Regulator gain and time constant [ Ka()  Ta(s) ]:"; exc "Exciter  [ Ke()  Te(s) ]:"; tgr "Transient gain reduction [ Tb(s)  Tc(s) ]:"; damp "Damping filter gain and time constant  [ Kf()  Tf(s)  ]:"; sat "Field saturation parameters [ A, B ]:"; lim "Regulator output limits and gain [ Efmin, Efmax (p.u.), Kp() ]:"; v0 "Initial values of terminal voltage  and field voltage [ Vt0 (pu) Vf0(pu) ] :"; Ts "Sample Time"
      mask help:
      | Implements an IEEE type 1 synchronous machine voltage regulator combined
      | to an exciter.
      |
      | The output of the block is the field voltage vfd, in p.u.,  to be applied to the Vf
      | Simulink input of a Synchronous Machine block.
      |
      | Connect the Vd and Vq measurements signals of the Synchronous Machine block
      | (signals 9 and 10)  to  the Vd and Vq inputs of the Excitation System block.
      mask init:
      | ka=reg(1);ta=reg(2);ke=exc(1);te=exc(2);tb=tgr(1);tc=tgr(2);kf=damp(1);tf=damp(2);efmin=lim(1);efmax=lim(2);a=sat(1);b=sat(2);kp=lim(3);
      | powericon('psbcallbacks',gcb,'Excitationsystem',1);
      mask Help: web(psbhelp);
  Gain : Gain  Gain=pTotal*1E9
  Mux : Mux  Inputs=2
  STG : powerlib/Machines/Steam Turbine and Governor  gentype=Tandem-compound (single mass)  reg1="[ 1  0.05    0 ]"  reg2="[ 0.001  0.15 ]"  reg3="[ -0.1  0.1  0  4.496 ]"  N=3600  turb1="[ 0  10   3.3   0.5   ]"  turb2="[   0   0.36    0.36   0.28   ]"  HA="[ 0.046  1.430  1.465   0.192 ]"  KA="[ 90.44  53.88  64.59   62.94  ]"  DA="[ 0.0115  0.3575  0.3663   0.0137  ]"  ini1=0.47  ini2=[0.779316,-31.4247]
  Terminator : Terminator
  Terminator1 : Terminator
  Terminator2 : Terminator
  wref : Constant
  Pm : Outport  InitialOutput=0
  Vf : Outport  Port=2  InitialOutput=0
  Peo_Delta : Outport  Port=3
  tag scope: P_G1=global, Q_G1=global, Wm_G1=global
  wires:
  m/1 -> Bus Selector/1
  "Delta w PSS (Kundur) "/1(Vstab) -> EXCITATION/4(vstab)
  STG/1 -> Terminator2/1
  STG/2 -> Terminator1/1
  STG/4 -> Pm/1
  STG/3 -> Terminator/1
  EXCITATION/1(Vf) -> Vf/1
  Vref/1 -> EXCITATION/1(vref)
  Pref/1 -> STG/2
  wref/1 -> STG/1
  Mux/1 -> Peo_Delta/1
  Gain/1 -> Mux/1
  Bus Selector/2 -> EXCITATION/3(vq)  "<Stator voltage  vq (pu)>"
  Bus Selector/1 -> EXCITATION/2(vd)  "<Stator voltage  vd (pu)>"
  Bus Selector/3 -> STG/4  "<Rotor angle deviation  d_theta (rad)>"
  Bus Selector/5 -> "Delta w PSS (Kundur) "/1(In)  "<Rotor speed deviation  dw (pu)>"
  Bus Selector/6 -> Mux/2  "<Load angle   delta  (deg)>"
  Bus Selector/7 -> [P_G1], Gain/1  "<Output active power   Peo (pu)>"
  Bus Selector/4 -> [Wm_G1], STG/3  "<Rotor speed  wm  (pu)>"
  Bus Selector/8 -> [Q_G1]  "<Output reactive power  Qeo (pu)>"

== system IEEE39bus/SS_WestSystem2/GT 2- Slack/Load 31/Load 31 ==
  Vabc : Inport
  Load shedding : Subsystem
  PLL1 : powerlib_meascontrol/PLL/PLL (3ph)  Fmin=45  Par_Init=[41.7 50]  ParK=[60 1400]  TcD=1e-4  MaxRateChangeFreq=12  FilterCutOffFreq=25  Ts=Ts  AGC=on
  Terminator1 : Terminator
  Load Power : Outport
  wires:
  PLL1/1 -> Load shedding/1(Local f)
  Vabc/1 -> PLL1/1
  PLL1/2 -> Terminator1/1
  Load shedding/1(Load Power) -> Load Power/1

== system IEEE39bus/SS_WestSystem1/GT 1 /The Electric Power Grid/M1TurbineRegulators/Delta w PSS (Kundur)  ==
  note: The simulink model of the Generic Power
      | System Stabilizer can be found in the
      | Continuous and Discrete libraries
      | of powerlib_models.
  In : Inport
  Source : Subsystem  mask(Generic PSS){Tsensor=Tsensor, K=K, Twashout=Twashout, Tleadlag1=Tleadlag1, Tleadlag2=Tleadlag2, VSlimits=VSlimits, Vinit=Vinit, Plot_On=off, MagdB_On=on, FreqRange=logspace(-2,2,500), Ts=Ts}
      mask prompts: Tsensor "Sensor time constant:"; K "Gain:"; Twashout "Wash-out time constant:"; Tleadlag1 "Lead-lag #1 time constants: [ Tnum Tden ]"; Tleadlag2 "Leag-lag #2 time constants: [ Tnum Tden ]"; VSlimits "Output limits: [ VSmin VSmax ]"; Vinit "Initial input:"; Plot_On "Plot frequency response"; MagdB_On "Magnitude in dB"; FreqRange "Frequency range (Hz):"
      mask help:
      | This block implements a generic Power System Stabilizer (PSS).
      |
      | Input (In): Synchronous machine speed deviation with respect to nominal (dw in pu) or acceleration power (Pa=Pm-Pe in pu).
      | Output (VS): stabilization voltage (pu).
      |
      | Look under mask to see how the various transfer functions are connected.
      mask init:
      | T1n=Tleadlag1(1);
      | T1d=Tleadlag1(2);
      | T2n=Tleadlag2(1);
      | T2d=Tleadlag2(2);
      | %
      | if Plot_On==1,
      | % Compute global system (sysG):
      | numS=[1];
      | denS=[Tsensor 1];
      | sysS=tf(numS,denS);
      | numW=[Twashout 0];
      | denW=[Twashout 1];
      | sysW=tf(numW,denW);
      | numL1=[T1n 1];
      | denL1=[T1d 1];
      | sysL1=tf(numL1,denL1);
      | numL2=[T2n 1];
      | denL2=[T2d 1];
      | sysL2=tf(numL2,denL2);
      | sysG=sysS*K*sysW*sysL1*sysL2;
      | %
      | % Plot response:
      | w=2*pi*FreqRange;
      | [Mag,Pha]=bode(sysG,w);
      | subplot(2,1,1)
      | if  MagdB_On==1,
      | Y= 20*log10(squeeze(Mag)) ;
      | strLabel='dB';
      | else
      | Y=squeeze(Mag);
      | strLabel='pu/pu';
      | end
      | %
      | semilogx(FreqRange,Y)
      | ylabel(strLabel);grid;
      | title('PSS Frequency Response');
      | subplot(2,1,2);
      | semilogx(FreqRange,rem(squeeze(Pha),360))
      | ylabel('Degrees');grid;
      | xlabel('Frequency (Hz)');
      | end
      mask Callback Plot_On: parametres=get_param(gcb,'MaskValues');p8=parametres{8};if strcmp(p8,'on');param9='on';param10='on';else;param9='off';param10='off';end;visible={'on','on','on','on','on','on','on','on',param9,param10,'on'};set_param(gcb,'MaskVisibilities',visible)
  Vstab : Outport  InitialOutput=0
  wires:
  Source/1(VS) -> Vstab/1
  In/1 -> Source/1(In)

== system IEEE39bus/SS_WestSystem1/GT 1 /The Electric Power Grid/M1TurbineRegulators/EXCITATION ==
  note: The simulink model of the Excitation system
      | can be found in the Continuous and Discrete
      | libraries of powerlib_models.
  vref : Inport
  vd : Inport  Port=2
  vq : Inport  Port=3
  vstab : Inport  Port=4
  Source : Subsystem  AncestorBlock=powerlib_models/Discrete/Excitation_System  mask(Discrete Excitation System){tr=tr, reg=reg, exc=exc, tgr=tgr, damp=damp, sat=sat, lim=lim, v0=v0, Ts=Ts}
      mask prompts: tr "Low-pass filter time constant Tr(s):"; reg "Regulator gain and time constant [ Ka()  Ta(s) ]:"; exc "Exciter  [ Ke()  Te(s) ]:"; tgr "Transient gain reduction [ Tb(s)  Tc(s) ]:"; damp "Damping filter gain and time constant  [ Kf()  Tf(s)  ]:"; sat "Field saturation parameters [ A, B ]:"; lim "Regulator output limits and gain [ Efmin, Efmax (p.u.), Kp() ]:"; v0 "Initial values of terminal voltage  and field voltage [ Vt0 (pu) Vf0(pu) ] :"; Ts "Sample time:"
      mask help:
      | Implements an discrete IEEE type 1 synchronous machine voltage regulator combined to an exciter. This block uses the dq components of terminal voltage (Synchronous Machine block, measurement ouputs 9 and 10).
      |
      | 1st input: desired stator terminal voltage (p.u.);
      | 2nd input: vd component of the terminal voltage (p.u.);
      | 3rd input: vq component of the terminal voltage (p.u.);
      | 4th input: stabilization voltage from user-supplied
      |                  power system stabilizer (p.u.);
      |
      | output: field voltage vfd to be applied to the
      |              Synchronous Machine block's 2nd input (p.u.).
      mask init:
      | ka=reg(1);ta=reg(2);ke=exc(1);te=exc(2);tb=tgr(1);tc=tgr(2);kf=damp(1);tf=damp(2);efmin=lim(1);efmax=lim(2);a=sat(1);b=sat(2);kp=lim(3);
      | if te==0,
      | te=1e-6;
      | end
      mask Help: web(psbhelp);
  Vf : Outport  InitialOutput=0
  wires:
  Source/1(Vf) -> Vf/1
  vref/1 -> Source/1(vref)
  vd/1 -> Source/2(vd)
  vq/1 -> Source/3(vq)
  vstab/1 -> Source/4(vstab)

== system IEEE39bus/SS_WestSystem2/GT 2- Slack/Load 31/Load 31/Load shedding ==
  Local f : Inport
  9.2MW->7.75MW : Step  Time=900  Before=[0.092e8 4.6e6]  After=[0.082763e8 4.6e6]  SampleTime=0
  Load shedding table : Lookup_n-D  NumberOfTableDimensions=1  BreakpointsForDimension1=[ 48.00 48.1 48.2 48.4 48.6 48.8 49]  Table=[ 0.5 0.55 0.65 0.75 0.85 0.95 1]  InterpMethod=Flat  InternalRulePriority=Speed  RndMeth=Simplest  InputSameDT=on
  Product : Product
  Load Power : Outport
  wires:
  Local f/1 -> Load shedding table/1
  Product/1 -> Load Power/1
  9.2MW->7.75MW/1 -> Product/2
  Load shedding table/1 -> Product/1
